simulink model "SimulateurNL_Pont_Cmd_Kw"  (R2022b)
settings: Solver=VariableStepAuto  StartTime=0.0  StopTime=30  MaxStep=0.001  RelTol=1e-3
values from neighbouring files (symbols this model uses):
  f = 7.25e-5    (= 7.25e-05)    [code.m]
  g = 9.81    [code.m]
  J = 3.9e-6    (= 3.9e-06)    [code.m]
  K_w = place(Aa,Ba,vp)    [code.m]
  Kfi = 4.77    [code.m]
  Ki = 5    [code.m]
  Komga = 0.02    [code.m]
  Kteta = 0.875    [code.m]
  Lm = 0.2e-3    (= 0.0002)    [code.m]
  N = 17    [Validation_param_pend.m]    (also in code.m)
  r = 0.022    [Validation_param_pend.m]    (also in code.m)
  Rm = 2.25    [code.m]
  Te = 0.002    [code.m]
  Te1 = 0.100    (= 0.1)    [code.m]    (also in matlab.mat = 0)
undefined symbols (not defined in the file or in its folder): DiscIntNeverNeededParam
libraries: simulink_extras x1
settings Model: Creator=Godoy  LastModifiedBy=corentinvenet
settings SolverCC: AlgebraicLoopSolver=TrustRegion
settings DataIOCC: ReturnWorkspaceOutputs=off
settings DebuggingCC: UnconnectedInputMsg=warning  UnconnectedOutputMsg=warning  UnconnectedLineMsg=warning  SFMachineParentedDataDiag=warning  ArithmeticOperatorsInVariantConditions=warning
settings ModelReferenceCC: EnableRefExpFcnMdlSchedulingChecks=on
settings SFSimCC: CustomCodeUndefinedFunction=UseInterfaceOnly

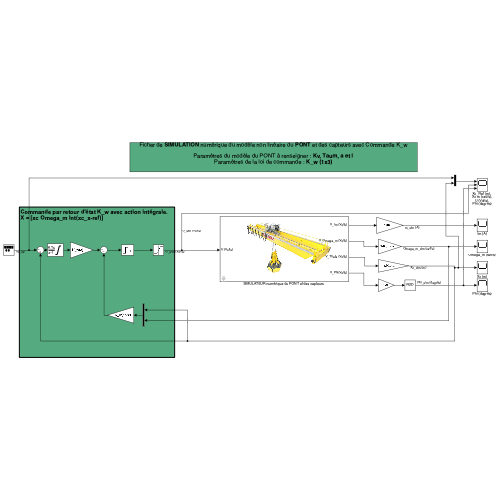
[thumbnail: Simulink's stored preview of the top-level diagram]
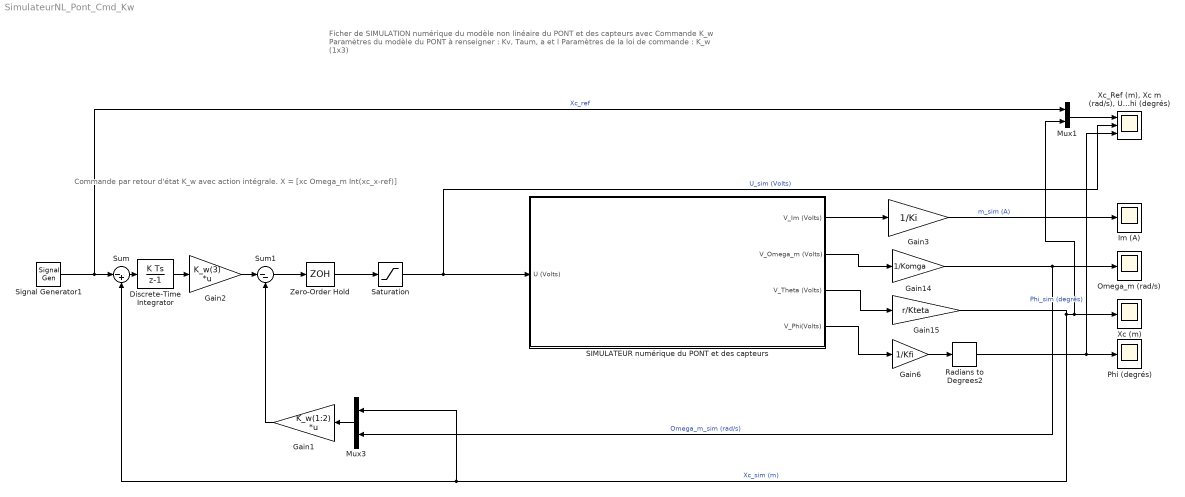
== system SimulateurNL_Pont_Cmd_Kw ==
  note: Commande par retour d'état K_w avec action intégrale.
      | X = [xc Omega_m Int(xc_x-ref)]
  note: Ficher de SIMULATION numérique du modèle non linéaire du PONT et des capteurs avec Commande K_w
      |
      | Paramètres du modèle du PONT à renseigner : Kv, Taum, a et l
      | Paramètres de la loi de commande : K_w (1x3)
  Discrete-Time Integrator : DiscreteIntegrator  SampleTime=Te  LimitOutput=on  UpperSaturationLimit=10  LowerSaturationLimit=-10  ICPrevOutput=DiscIntNeverNeededParam  ICPrevScaledInput=DiscIntNeverNeededParam
  Gain1 : Gain  Gain=K_w(1:2)  Multiplication=Matrix(K*u)
  Gain14 : Gain  Gain=1/Komga
  Gain15 : Gain  Gain=r/Kteta
  Gain2 : Gain  Gain=K_w(3)  Multiplication=Matrix(K*u)
  Gain3 : Gain  Gain=1/Ki
  Gain6 : Gain  Gain=1/Kfi
  Im (A) : Scope
  Mux1 : Mux  Inputs=2
  Mux3 : Mux  Inputs=2
  Omega_m (rad/s) : Scope
  Phi (degrés) : Scope
  Radians to Degrees2 : simulink_extras/Transformations/Radians to Degrees
  "SIMULATEUR numérique du PONT et des capteurs " : Subsystem  mask{Kv=43.3, Taum=0.035, a=0.0487, l=0.2687}
      mask prompts: l "longueur l (m)"
      mask Display: image('$imagefile'); % Use "Edit Image" on toolstrip to change.
  Saturation : Saturate  UpperLimit=9.99  LowerLimit=-9.99
  Signal Generator1 : SignalGenerator  WaveForm=square  Amplitude=0.15  Frequency=0.1
  Sum : Sum  Inputs=|-+
  Sum1 : Sum  Inputs=|--
  Xc (m) : Scope
  "Xc_Ref (m), Xc m (rad/s), U (Volts), Phi (degrés)" : Scope  NumInputPorts=3
  Zero-Order Hold : ZeroOrderHold  SampleTime=Te1
  wires:
  Gain14/1 -> Mux3/2, Omega_m (rad/s)/1  "Omega_m_sim (rad/s)"
  "SIMULATEUR numérique du PONT et des capteurs "/3(V_Theta (Volts)) -> Gain15/1
  "SIMULATEUR numérique du PONT et des capteurs "/4(V_Phi(Volts)) -> Gain6/1
  "SIMULATEUR numérique du PONT et des capteurs "/2(V_Omega_m (Volts)) -> Gain14/1
  Radians to Degrees2/1 -> Phi (degrés)/1, "Xc_Ref (m), Xc m (rad/s), U (Volts), Phi (degrés)"/3  "Phi_sim (degrés)"
  "SIMULATEUR numérique du PONT et des capteurs "/1(V_Im (Volts)) -> Gain3/1
  Gain6/1 -> Radians to Degrees2/1
  Gain3/1 -> Im (A)/1  "m_sim (A)"
  Saturation/1 -> "SIMULATEUR numérique du PONT et des capteurs "/1(U (Volts)), "Xc_Ref (m), Xc m (rad/s), U (Volts), Phi (degrés)"/2  "U_sim (Volts)"
  Discrete-Time Integrator/1 -> Gain2/1
  Zero-Order Hold/1 -> Saturation/1
  Gain1/1 -> Sum1/2
  Gain15/1 -> Mux3/1, Sum/2, Mux1/2, Xc (m)/1  "Xc_sim (m)"
  Mux3/1 -> Gain1/1
  Gain2/1 -> Sum1/1
  Sum/1 -> Discrete-Time Integrator/1
  Signal Generator1/1 -> Mux1/1, Sum/1  "Xc_ref"
  Mux1/1 -> "Xc_Ref (m), Xc m (rad/s), U (Volts), Phi (degrés)"/1
  Sum1/1 -> Zero-Order Hold/1

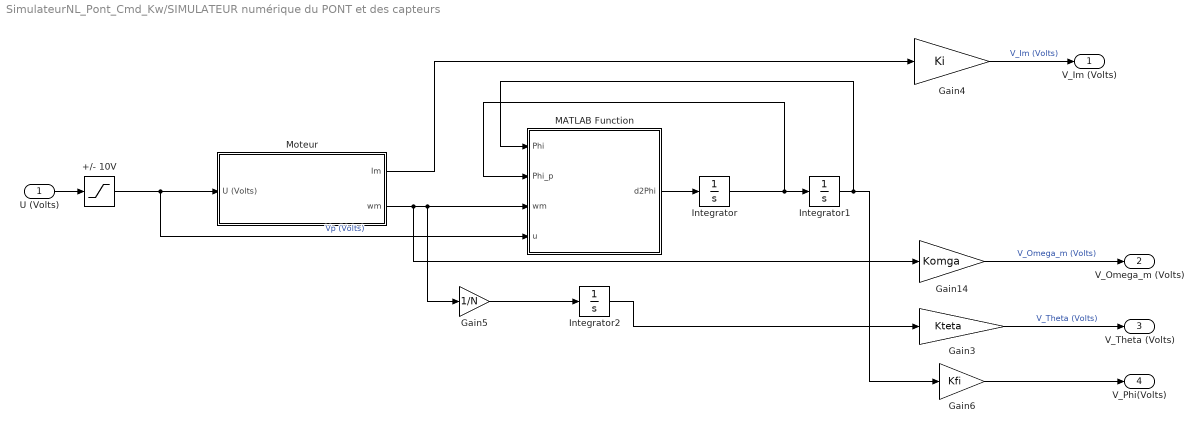
== system SimulateurNL_Pont_Cmd_Kw/SIMULATEUR numérique du PONT et des capteurs  ==
  U (Volts) : Inport
  +/- 10V : Saturate  UpperLimit=10  LowerLimit=-10
  Gain14 : Gain  Gain=Komga
  Gain3 : Gain  Gain=Kteta
  Gain4 : Gain  Gain=Ki
  Gain5 : Gain  Gain=1/N
  Gain6 : Gain  Gain=Kfi
  Integrator : Integrator
  Integrator1 : Integrator
  Integrator2 : Integrator
  MATLAB Function : MATLAB Function  TreatAsAtomicUnit=on
  Moteur : Subsystem
  V_Im (Volts) : Outport
  V_Omega_m (Volts) : Outport  Port=2
  V_Theta (Volts) : Outport  Port=3
  V_Phi(Volts) : Outport  Port=4
  wires:
  U (Volts)/1 -> +/- 10V/1
  Gain14/1 -> V_Omega_m (Volts)/1  "V_Omega_m (Volts)"
  Moteur/2(wm) -> Gain14/1, Gain5/1, MATLAB Function/3(wm)
  Gain5/1 -> Integrator2/1
  MATLAB Function/1(d2Phi) -> Integrator/1
  Moteur/1(Im) -> Gain4/1
  Integrator/1 -> MATLAB Function/2(Phi_p), Integrator1/1
  Integrator1/1 -> Gain6/1, MATLAB Function/1(Phi)
  Gain6/1 -> V_Phi(Volts)/1
  Integrator2/1 -> Gain3/1
  Gain4/1 -> V_Im (Volts)/1  "V_Im (Volts)"
  Gain3/1 -> V_Theta (Volts)/1  "V_Theta (Volts)"
  +/- 10V/1 -> MATLAB Function/4(u), Moteur/1(U (Volts))  "Vp (Volts)"

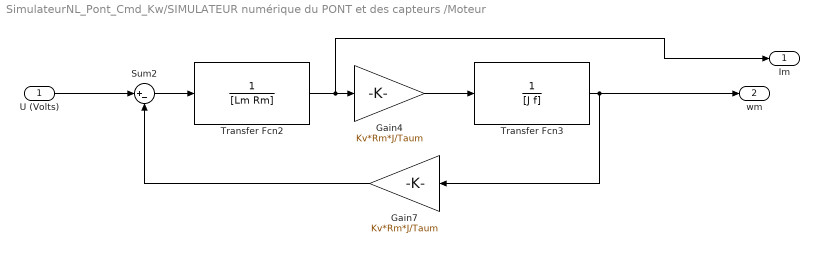
== system SimulateurNL_Pont_Cmd_Kw/SIMULATEUR numérique du PONT et des capteurs /Moteur ==
  U (Volts) : Inport
  Gain4 : Gain  Gain=Kv*Rm*J/Taum
  Gain7 : Gain  Gain=Kv*Rm*J/Taum
  Sum2 : Sum  Inputs=|+-
  Transfer Fcn2 : TransferFcn  Denominator=[Lm Rm]
  Transfer Fcn3 : TransferFcn  Denominator=[J f]
  Im : Outport
  wm : Outport  Port=2
  wires:
  U (Volts)/1 -> Sum2/1
  Gain7/1 -> Sum2/2
  Transfer Fcn2/1 -> Gain4/1, Im/1
  Sum2/1 -> Transfer Fcn2/1
  Gain4/1 -> Transfer Fcn3/1
  Transfer Fcn3/1 -> Gain7/1, wm/1

== matlab function SimulateurNL_Pont_Cmd_Kw/SIMULATEUR numérique du PONT et des capteurs /MATLAB Function ==
  data: Phi input; Phi_p input; wm input; u input; d2Phi output size=1; r parameter; N parameter; l parameter; a parameter; Taum parameter; Kv parameter; g parameter
function d2Phi = fcn(Phi, Phi_p, wm, u, r, N, l, a, Taum, Kv, g)

d2Phi=(-r/N*cos(Phi)*(-1/Taum*wm+Kv/Taum*u)-g*sin(Phi) -a*Phi_p)/l;
